simulink model "Water_Tank_volume_management_system"  (R2024b)
settings: Solver=VariableStepAuto  StartTime=0.0  StopTime=inf  RelTol=1e-3
settings Model: Creator=rohan  LastModifiedBy=rohan

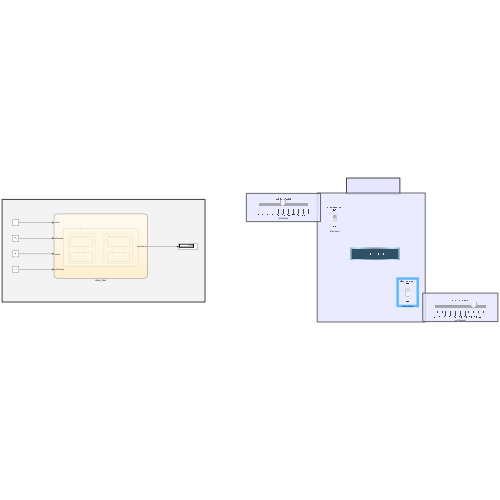
[thumbnail: Simulink's stored preview of the top-level diagram]
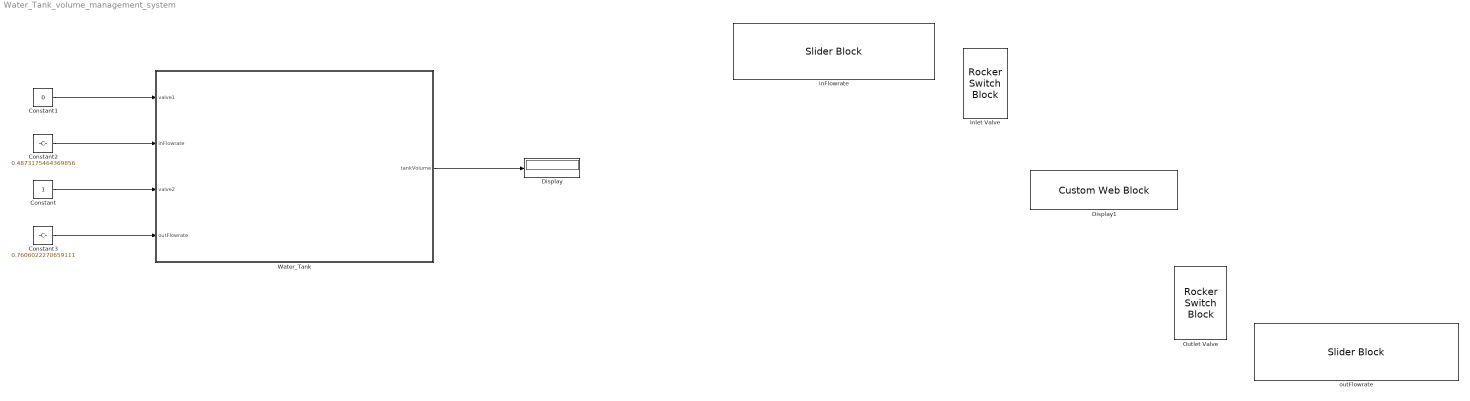
== system Water_Tank_volume_management_system ==
  Constant : Constant
  Constant1 : Constant  Value=0
  Constant2 : Constant  Value=0.4873175464369856
  Constant3 : Constant  Value=0.7606022270659111
  Display : Display
  Display1 : CustomWebBlock  LabelPosition=Hide  ShowInitialText=on  Configuration="{\"components\":[{\"name\":\"DisplayComponent\",\"settings\":{\"bold\":false,\"font\":\"DSEG7 Classic\",\"fontColor\":[255,255,200],\"fontSize\":\"14\",\"format\":\"short\",\"formatString\":\"%d\",\"italic\":false,\"position\":[0,0,1,1],\"underline\":false}},{\"name\":\"BackgroundImageComponent\",\"settings\":{\"image\":{\"size\":[300,80],\"src\":\"data:image\\/svg+xml;base64,PHN2ZyBpZD0iZnJhbWUiIHhtbG5zPSJodHRwOi8vd3d3LnczLm9yZy8yMDAwL3N2ZyIgeG1sbnM6eGxpbms9Imh0dHA6Ly93d3cudzMub3JnLzE5OTkveGxpbmsiIHZpZXdCb3g9IjAgMCAzODAgMTAxIj48ZGVmcz48c3R5bGU+LmNscy0xe2ZpbGw6IzAwMmI0Mjt9LmNscy0ye2ZpbGw6IzQyNzA4Mjt9LmNscy0ze2ZpbGw6dXJsKCNyYWRpYWwtZ3JhZGllbnQpO308L3N0eWxlPjxyYWRpYWxHcmFkaWVudCBpZD0icmFkaWFsLWdyYWRpZW50IiBjeD0iMTkwIiBjeT0iNTAuNSIgcj0iMjY5LjIxIiBncmFkaWVudFVuaXRzPSJ1c2VyU3BhY2VPblVzZSI+PHN0b3Agb2Zmc2V0PSIwLjAxIiBzdG9wLWNvbG9yPSIjM2U0ZjU4Ii8+PHN0b3Agb2Zmc2V0PSIwLjA2IiBzdG9wLWNvbG9yPSIjNDQ1NzYxIi8+PHN0b3Agb2Zmc2V0PSIwLjE1IiBzdG9wLWNvbG9yPSIjNTU2YTc2Ii8+PHN0b3Agb2Zmc2V0PSIwLjI1IiBzdG9wLWNvbG9yPSIjNmQ4ODk1Ii8+PHN0b3Agb2Zmc2V0PSIwLjM4IiBzdG9wLWNvbG9yPSIjOGZiMmMzIi8+PHN0b3Agb2Zmc2V0PSIwLjUyIiBzdG9wLWNvbG9yPSIjYjZlNGZhIi8+PHN0b3Agb2Zmc2V0PSIxIiBzdG9wLWNvbG9yPSIjMTU0NjU3Ii8+PC9yYWRpYWxHcmFkaWVudD48L2RlZnM+PGcgaWQ9IkxheWVyXzIiIGRhdGEtbmFtZT0iTGF5ZXIgMiI+PGcgaWQ9IkxheWVyXzEtMiIgZGF0YS1uYW1lPSJMYXllciAxLTIiPjxyZWN0IGlkPSJyZWN0MTAzNiIgY2xhc3M9ImNscy0xIiB4PSIxMSIgeT0iMTEiIHdpZHRoPSIzNTgiIGhlaWdodD0iNzkiLz48cGF0aCBpZD0icGF0aDEwMzgiIGNsYXNzPSJjbHMtMiIgZD0iTTgsOFY5M0gzNzJWOFpNMzY5LDkwSDExVjExSDM2OVoiLz48cGF0aCBpZD0icGF0aDEwNDAiIGNsYXNzPSJjbHMtMyIgZD0iTTAsMFYxMDFIMzgwVjBaTTM3Miw5M0g4VjhIMzcyWiIvPjwvZz48L2c+PC9zdmc+\",\"srcOrientation\":\"Right\"},\"position\":[0,0,1,1],\"scaleMode\":\"0\"}},{\"name\":\"ForegroundImageComponent\",\"settings\":{\"angle\":0,\"image\":{\"size\":[0,0],\"src\":\"default\"},\"isForeground\":1,\"position\":[0,0,1,1],\"scaleMode\":\"0\"}}],\"settings\":{\"BindingType\":\"signal\",\"aspectRatio\":1.032258064516129,\"backgroundColor\":[0,0,0,\"1\"],\"backgroundOffset\":0.14,\"backgroundOpacity\":1,\"fixedAspectRatio\":\"on\",\"showBackgroundColor\":false,\"value\":0,\"version\":\"R2023b\"},\"type\":\"Display\"}"
  Inlet Valve : RockerSwitchBlock
      settings: Values={{'Off', 'On'}, [0 1]}
  Outlet Valve : RockerSwitchBlock
      settings: Values={{'Off', 'On'}, [0 1]}
  Water_Tank : Stateflow chart  TreatAsAtomicUnit=on
      settings: PortSchema="{\"entries\":[{\"content\":{\"sides\":[{\"content\":{\"connectorIds\":[\"In3\",\"In2\",\"In4\",\"In1\"]},\"type\":\"ConnectorPlacement.EquallySpacedRectSide\",\"uuid\":\"e648238b-3503-4683-b81e-6d8918cd4221\"},{\"content\":{\"connectorIds\":[\"Out1\"],\"side\":\"RIGHT\"},\"type\":\"ConnectorPlacement.EquallySpacedRectSide\",\"uuid\":\"ba9fd920-e1a8-439a-9093-b2c0a64093ff\"},{\"content\":{\"side\":\"TOP\"},\"type\":\"ConnectorPlacement.EquallySpacedRectSide\",\"uuid\":\"d79003d1-8058-4701-bc52-c464771b0f52\"}]},\"type\":\"ConnectorPlacement.EquallySpacedConnector\",\"uuid\":\"e1f4e958-29da-49b2-ab5f-02b0150a0b53\"}],\"packageUris\":[\"http://schema.mathworks.com/mf0/Connector/R2020b\"],\"version\":\"1.0\"}"
  inFlowrate : SliderBlock  ScaleMax=1
  outFlowrate : SliderBlock  ScaleMax=1
  wires:
  Constant/1 -> Water_Tank/4(valve2)
  Constant1/1 -> Water_Tank/3(valve1)
  Constant2/1 -> Water_Tank/2(inFlowrate)
  Constant3/1 -> Water_Tank/1(outFlowrate)
  Water_Tank/1(tankVolume) -> Display/1

== stateflow chart Water_Tank_volume_management_system/Water_Tank ==
  state waterTank
    % fill and empty are in dotted lines because both the operations are occuring parallely, i.e. a tank can be filled and emptied at the same time.
    % To set two states to occurs parallely, right-click inside the main state(waterTank in this case) -> Decomposition -> Parallel (AND)
    state fill [parallel]
      settings: executionOrder=1
      state valve1_close
      state valve2_open
        tankVolume=min((tankVolume+inFlowrate),100);
      (default) -> valve1_close
      valve1_close -> waterTank.fill.valve2_open : [valve1==1 &&...
          | tankVolume<=100]
      waterTank.fill.valve2_open -> valve1_close : [valve1==0||...
          | tankVolume>=100]
    state empty [parallel]
      settings: executionOrder=2
      state valve2_close
      state valve2_open
        tankVolume=max((tankVolume-outFlowrate),0);
      (default) -> valve2_close
      valve2_close -> waterTank.empty.valve2_open : [valve2==1 &&...
          | tankVolume>=0]
      waterTank.empty.valve2_open -> valve2_close : [valve2==0||...
          | tankVolume<=0]
  (default) -> waterTank
  data: outFlowrate input; inFlowrate input; valve1 input; valve2 input; tankVolume output [0..100] =0
